simulink model "Monorail_Auxiliary_Power_Unit"  (R2021b)
settings: Solver=ode1  StartTime=0.0  StopTime=2.00  FixedStep=1e-06  MaxStep=1e-4  RelTol=1e-3
InitFcn:
  | %Input
  | V_supply_max = 910;
  | V_supply_min = 490;
  | V_supply_nom = 750;
  | R_supply = 1e-06;
  | L_in = 0.5e-03;
  | C_in = 215e-06;
  | R_Precharge = 1;
  | 
  | %PSFB_Voltage_Control
  | t_psfb_on = 0.05;
  | f_sw = 10e03;
  | V_dc_ref = 700;
  | V_dc_init = 450;
  | V_bat_ref = 24;
  | V_bat_init = 14;
  | Count_prd = 5000;
  | Half_prd = 2500;
  | Half_prd_fix = 2700;
  | Half_prd_var = 2300;
  | t_softstart = 100e-03;
  | Scale_factor_High = 1/737;
  | Scale_factor_Low = 1/48;
  | Kp_psfb = 2;
  | Ki_psfb =20;
  | Kp_feed = 0.00001;
  | PI_max = 1;
  | PI_min = 0;
  | t_enable = 1e-03;
  | Dead_prd = 1e-03
  | 
  | %PSFB_Current_Control
  | Scale_factor_i = 1/800;
  | I_cnst = 450;
  | I_over = 460;
  | Kp_psfb_i = 10;
  | Ki_psfb_i = 20;
  | 
  | %HF_Transformer
  | P_txf = 50e03;
  | f_txf = 10e03;
  | V_pri_txf = 1e03;
  | V_sec_high_txf = 720;
  | V_sec_low_txf = 27;
  | 
  | %DC_Link
  | L_filt = 1e-03;
  | C_filt = 215e-06;
  | R_Bleeder_700V = 0.5e03;
  | R_Bleeder_24V = 1e03
  | 
  | %Inverter_Control
  | t_inv_on = 1.5;
  | f_fund = 50;
  | V_phase_ref = 240;
  | Scale_factor_inv = 1/50e03;
  | Kp_inv = 0.05;
  | Ki_inv = 0.1;
  | PI_inv_max = 1;
  | PI_inv_min = -1;
  | I_Line_ref = 35;
  | Scale_factor_Iinv = 1/1e03;
  | Iinvov = 40;
  | Kp_Iinv = 0.05;
  | Ki_Iinv = 0.1;
  | t_dead = 2e-06;
  | 
  | %Inverter_Filter
  | L_sin_filt = 0.85e-03;
  | C_sin_filt = 30e-06;
  | 
  | %Zigzag
  | P_zigzag = 2.5e3;
  | f_zigzag = 50;
  | V_zigzag = 415;
  | 
  | %Load
  | R_load_750V = 6;
  | L_load_750V = 14.3e-03;
  | R_overload_750V = 6;
  | L_overload_750V = 14.3e-03;
  | t_overload_750V = 5;
  | R_load_24V = 53e-03;
  | R_overload_24V = 168e-03;
  | t_overload_24V = 5;
  | R_load_si = 24;
  | t_load_si = 10;
undefined symbols (not defined in the file): Ion, Lithium
libraries: spsSeriesRLCBranchLib x35, spsIGBTDiodeLib x14, spsDiodeLib x13, spsMeanLib x11, spsBreakerLib x9, spsVoltageMeasurementLib x9, simulink x8, spsRMSLib x8, spsCurrentMeasurementLib x6, dspfdesign x6, spsabctodq0Lib x4, spsLinearTransformerLib x2
(part 1 of 3)
settings Model: ModifiedByFormat=Sourjya_Mondal  Creator=Sourjya_Mondal  LastModifiedBy=Sourjya_Mondal
settings SolverCC: AlgebraicLoopSolver=TrustRegion  AutoInsertRateTranBlk=on
settings DataIOCC: ReturnWorkspaceOutputs=off
settings OptimizationCC: LifeSpan=inf
settings DebuggingCC: SFUnexpectedBacktrackingDiag=warning  SFNoUnconditionalDefaultTransitionDiag=warning  SFExecutionAtInitializationDiag=none  SFMachineParentedDataDiag=warning  ArithmeticOperatorsInVariantConditions=warning
settings SFSimCC: SimUseLocalCustomCode=off  CustomCodeUndefinedFunction=UseInterfaceOnly
settings RTWCC: RTWUseLocalCustomCode=off
settings CodeAppCC: StateflowObjectComments=on
settings GRTTargetCC: TargetLangStandard=C89/C90 (ANSI)
settings ConfigComp: CovMetricSettings=dw  CovSaveCumulativeToWorkspaceVar=on  CovSaveSingleToWorkspaceVar=on  CovExternalEMLEnable=off
settings SimscapeCC: SimscapeNormalizeSystem=off

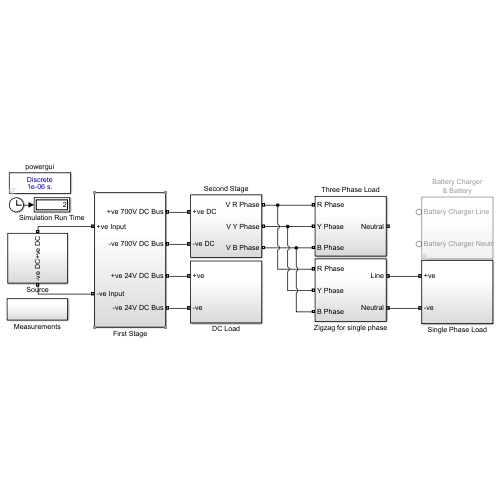
[thumbnail: Simulink's stored preview of the top-level diagram]
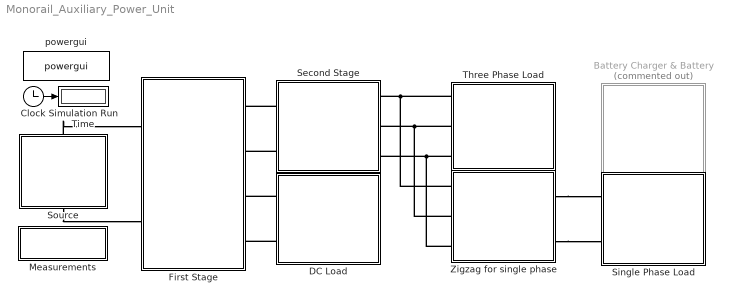
== system Monorail_Auxiliary_Power_Unit ==
  Battery Charger & Battery : Subsystem  Commented=on
  Clock : Clock
  DC Load : Subsystem
  First Stage : Subsystem
  Measurements : Subsystem
  Second Stage : Subsystem
  Simulation Run Time : Display
  Single Phase Load : Subsystem
  Source : Subsystem
  Three Phase Load : Subsystem
  Zigzag for single phase : Subsystem
  powergui : spspowerguiLib/powergui  Priority=1  SimulationMode=Discrete  SampleTime=1e-06  frequency=60  Iterations=50  frequencyindice=0  Pbase=100e6  ErrMax=1e-4  UnitsV=kV  UnitsW=MW  buscounter=0  FunctionMessages=off  echomessages=off  EnableUseOfTLC=off  CurrentSourceSwitches=off  DisableSnubberDevices=off  DisableRonSwitches=off  DisableVfSwitches=off  DisplayEquations=off  AutomaticDiscreteSolvers=off  SolverType=Tustin/Backward Euler (TBE)  Interpol=off  ExternalGateDelay=off  methode=off  Ts=100  x0status=blocks  SPID=on  SwTol=0  HookPort=off  NonlinearTolerance=1e-4  nMaxIteration=100  ContinueOnMaxIteration=off  RestoreLinks=warning  ResistiveCurrentMeasurement=off  Frange=[0:2:500]  Ylog=off  Xlog=on  ShowGrid=off  save=off  variable=ZData  structure=V_line  ZoomFFT=off  StartTime=0.1  cycles=5  DisplayStyle=1  fundamental=50  FreqAxis=off  MaxFrequency=10000  frequencyindicesteady=1  RmsSteady=1  display=off
  wires:
  Clock/1 -> Simulation Run Time/1
  connections:
  Source/LConn1 -- First Stage/LConn2
  Source/RConn1 -- First Stage/LConn1
  Second Stage/LConn1 -- First Stage/RConn1
  Second Stage/LConn2 -- First Stage/RConn2
  Three Phase Load/LConn1 -- Second Stage/RConn1 -- Zigzag for single phase/LConn1
  Three Phase Load/LConn3 -- Zigzag for single phase/LConn3 -- Second Stage/RConn3
  DC Load/LConn1 -- First Stage/RConn3
  DC Load/LConn2 -- First Stage/RConn4
  Three Phase Load/LConn2 -- Zigzag for single phase/LConn2 -- Second Stage/RConn2
  Zigzag for single phase/RConn1 -- Single Phase Load/LConn1
  Zigzag for single phase/RConn2 -- Single Phase Load/LConn2

== system Monorail_Auxiliary_Power_Unit/Battery Charger & Battery ==
  Battery : spsBatteryLib/Battery  BatType=Lithium-Ion  ShowTempParam=off  ThermalPreset=no  ShowAgeParam=off  NomV=24  NomQ=10  SOC=0  Batt_Tr=30  PresetModel=on  MaxQ=10  MinV=18  FullV=27.9357  Dis_rate=4.3478  R=0.024  Normal_OP=9.0435  expZone="[25.9293     0.491304]"  current=[6.5 13 32.5]  Units=Time  Tci=20  NomT=20  T2=-30  MaxQ2=4.8  FullV2=7.1  Normal_OP2=5.655  expZone2="[6.58           1]"  Rca=0.6  ti=2000  Dp=0  Neq0=0  Tsim=1e6  Ta1=25  Qeol=5.4*0.9  Reol=0.013333*1.2  Char_age=[2.3478, 3]  Dis_age=[2.3478, 10]  N1=1500  N2=10500  N3=1000  N4=1400  Ta2=45  N5=950
  Bus Selector : BusSelector  OutputSignals=Input Voltage (V),Input Current (A),Output Voltage (V),Output Current (A),Voltage limit (V),Current limit (A),Output KWh,Output Ah
  Bus Selector1 : BusSelector  OutputSignals=Voltage (V),Current (A),SOC (%)
  CCCV Battery Charger : electricdrivelib/Extra Sources/CCCV Battery Charger  Preset=Custom specifications  P_nom=800  s_type=1-phase AC  n_connect=off  eff_volt=240  in_freq=50  in_I_ripple=10  in_I_freq=1000  EFF_en=off  EFF_val=[0.627 0.803 0.855 0.871 0.872 0.864]  EFF_fu=[0.063 0.177 0.293 0.483 0.674 0.914]  THD_en=off  I_THD_val=[0.327 0.394 0.394 0.351 0.289 0.265]  I_THD_fu=[0.056 0.136 0.194 0.303 0.555 0.916]  H_DIST_rt=[0.199 1.297 0.328 0.029 0.416 0.200]  H_DIST_fr=[3 5 7 9 11 13]  PF_en=off  PF_val=[0.316 0.532 0.662 0.731 0.780 0.792]  PF_fu=[0.067 0.230 0.445 0.625 0.794 0.919]  Out_mode=Constant Current - Constant Voltage (CCCV)  DynInT=off  I_cst=10  V_cst=32  ABS_en=off  V_abs=142  ABS_end=Time based  ABS_time=3600  ABS_i=40  ripple=0.5  swF=1000  overshoot=1  stable_t=2  VoltComp=off  V_comp=-0.18  nom_temp=20
      settings: SourceProductBaseCode=PS
  Scope : Scope  NumInputPorts=8
  Scope1 : Scope  NumInputPorts=3
  Battery Charger Line : PMIOPort  Side=Left
  Battery Charger Neutral : PMIOPort  Port=2  Side=Left
  wires:
  Battery/1 -> Bus Selector1/1
  CCCV Battery Charger/1 -> Bus Selector/1
  Bus Selector/1 -> Scope/1  "<Input Voltage (V)>"
  Bus Selector/2 -> Scope/2  "<Input Current (A)>"
  Bus Selector/3 -> Scope/3  "<Output Voltage (V)>"
  Bus Selector/4 -> Scope/4  "<Output Current (A)>"
  Bus Selector/5 -> Scope/5  "<Voltage limit (V)>"
  Bus Selector/6 -> Scope/6  "<Current limit (A)>"
  Bus Selector/7 -> Scope/7  "<Output KWh>"
  Bus Selector/8 -> Scope/8  "<Output Ah>"
  Bus Selector1/1 -> Scope1/1, [VBat]  "<Voltage (V)>"
  Bus Selector1/2 -> [IBat], Scope1/2  "<Current (A)>"
  Bus Selector1/3 -> [Soc_Bt], Scope1/3  "<SOC (%)>"
  connections:
  Battery/LConn2 -- CCCV Battery Charger/RConn2
  CCCV Battery Charger/LConn2 -- Battery Charger Neutral/RConn1
  CCCV Battery Charger/LConn1 -- Battery Charger Line/RConn1
  Battery/LConn1 -- CCCV Battery Charger/RConn1

== system Monorail_Auxiliary_Power_Unit/DC Load ==
  Breaker : spsBreakerLib/Breaker  InitialState=0  SwitchingTimes="[1/60  5/60]"  External=on  BreakerResistance=0.01  SnubberResistance=1e6  SnubberCapacitance=inf  Measurements=None  MoreParameters=on  NoBreakLoop=off
      settings: SourceProductBaseCode=PS
  Enable : Step  Time=t_overload_24V  SampleTime=0
  Load 24V : spsSeriesRLCBranchLib/Series RLC Branch  LConnTagsString=__new0  RConnTagsString=__new0  BranchType=R  Resistance=R_load_24V  Inductance=1e-3  SetiL0=off  InitialCurrent=0  Capacitance=1e-6  Setx0=off  InitialVoltage=0  Measurements=None
  Overload 24V : spsSeriesRLCBranchLib/Series RLC Branch  LConnTagsString=__new0  RConnTagsString=__new0  BranchType=R  Resistance=R_overload_24V  Inductance=1e-3  SetiL0=off  InitialCurrent=0  Capacitance=1e-6  Setx0=off  InitialVoltage=0  Measurements=None
  +ve : PMIOPort  Side=Left
  -ve : PMIOPort  Port=2  Side=Left
  wires:
  Enable/1 -> Breaker/1
  connections:
  Load 24V/RConn1 -- -ve/RConn1 -- Overload 24V/RConn1
  Breaker/RConn1 -- Overload 24V/LConn1
  Load 24V/LConn1 -- +ve/RConn1 -- Breaker/LConn1

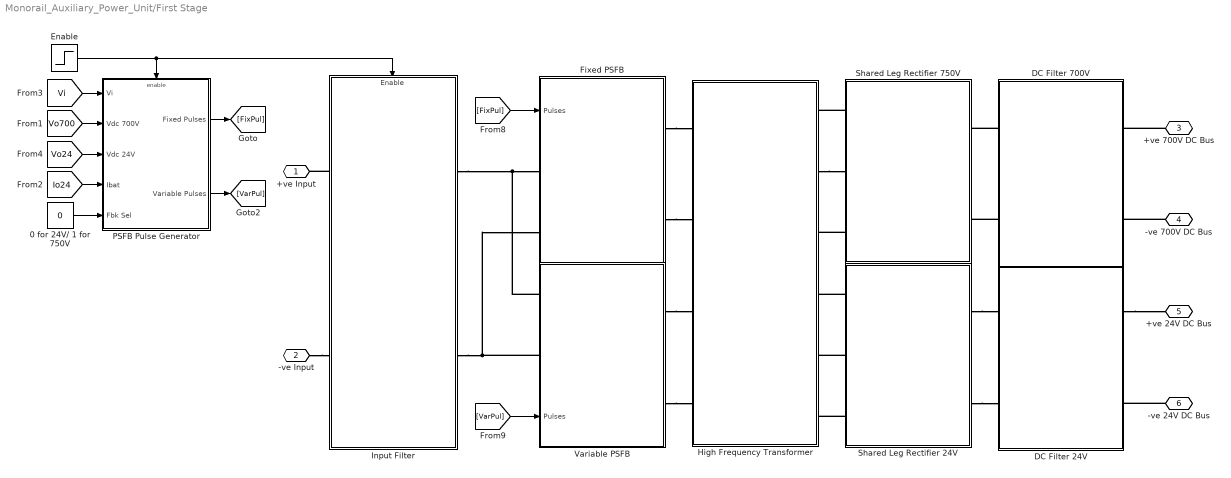
== system Monorail_Auxiliary_Power_Unit/First Stage ==
  0 for 24V/ 1 for 750V : Constant  Value=0
  DC Filter 24V : Subsystem
  DC Filter 700V : Subsystem
  Enable : Step  Time=t_psfb_on  SampleTime=0
  Fixed PSFB : Subsystem
  High Frequency Transformer : Subsystem
  Input Filter : Subsystem
      settings: PortSchema="{\"entries\":[{\"content\":{\"sides\":[{\"content\":{\"connectorIds\":[\"LConn1\",\"LConn2\"]},\"type\":\"ConnectorPlacement.EquallySpacedRectSide\",\"uuid\":\"355a31a2-ce4b-4446-9817-9663033cd28f\"},{\"content\":{\"connectorIds\":[\"RConn1\",\"RConn2\"],\"side\":\"RIGHT\"},\"type\":\"ConnectorPlacement.EquallySpacedRectSide\",\"uuid\":\"b1fa4b98-51e4-4b38-9334-3febb64d3166\"},{\"content\":{\"connectorIds\":[\"In1\"],\"side\":\"TOP\"},\"type\":\"ConnectorPlacement.EquallySpacedRectSide\",\"uuid\":\"3f1f76b0-45f3-4470-8606-701da3bcbe91\"}]},\"type\":\"ConnectorPlacement.EquallySpacedConnector\",\"uuid\":\"958f5b0f-2907-4940-ab6c-951926d8c97d\"}],\"packageUris\":[\"http://schema.mathworks.com/mf0/Connector/19700101\"],\"version\":\"1.0\"}"
  PSFB Pulse Generator : Subsystem
  Shared Leg Rectifier 24V : Subsystem
  Shared Leg Rectifier 750V : Subsystem
  Variable PSFB : Subsystem
      settings: PortSchema="{\"entries\":[{\"content\":{\"sides\":[{\"content\":{\"connectorIds\":[\"LConn1\",\"LConn2\",\"In1\"]},\"type\":\"ConnectorPlacement.EquallySpacedRectSide\",\"uuid\":\"164ee9a8-2883-4226-b641-75c923cc026a\"},{\"content\":{\"connectorIds\":[\"RConn1\",\"RConn2\"],\"side\":\"RIGHT\"},\"type\":\"ConnectorPlacement.EquallySpacedRectSide\",\"uuid\":\"3b4b1bb8-e497-4734-a92c-e609f39791cc\"},{\"content\":{\"connectorIds\":[],\"side\":\"TOP\"},\"type\":\"ConnectorPlacement.EquallySpacedRectSide\",\"uuid\":\"0bc5d7e7-4d54-414e-b6a1-3dfe739bfaa8\"}]},\"type\":\"ConnectorPlacement.EquallySpacedConnector\",\"uuid\":\"01def37e-b1d8-481f-9d3c-6964dbf0bd56\"}],\"packageUris\":[\"http://schema.mathworks.com/mf0/Connector/19700101\"],\"version\":\"1.0\"}"
  +ve Input : PMIOPort  Side=Left
  -ve Input : PMIOPort  Port=2  Side=Left
  +ve 700V DC Bus : PMIOPort  Port=3  Side=Right
  -ve 700V DC Bus : PMIOPort  Port=4  Side=Right
  +ve 24V DC Bus : PMIOPort  Port=5  Side=Right
  -ve 24V DC Bus : PMIOPort  Port=6  Side=Right
  wires:
  [FixPul] -> Fixed PSFB/1(Pulses)
  [VarPul] -> Variable PSFB/1(Pulses)
  0 for 24V/ 1 for 750V/1 -> PSFB Pulse Generator/5(Fbk Sel)
  PSFB Pulse Generator/1(Fixed Pulses) -> [FixPul]
  PSFB Pulse Generator/2(Variable Pulses) -> [VarPul]
  Enable/1 -> Input Filter/1(Enable), PSFB Pulse Generator/Enable
  [Vo24] -> PSFB Pulse Generator/3(Vdc 24V)
  [Vo700] -> PSFB Pulse Generator/2(Vdc 700V)
  [Io24] -> PSFB Pulse Generator/4(Ibat)
  [Vi] -> PSFB Pulse Generator/1(Vi)
  connections:
  Shared Leg Rectifier 24V/LConn2 -- High Frequency Transformer/RConn5
  Shared Leg Rectifier 24V/LConn1 -- High Frequency Transformer/RConn4
  +ve 700V DC Bus/RConn1 -- DC Filter 700V/RConn1
  Shared Leg Rectifier 24V/RConn1 -- DC Filter 24V/LConn1
  DC Filter 700V/LConn2 -- Shared Leg Rectifier 750V/RConn2
  Shared Leg Rectifier 24V/RConn2 -- DC Filter 24V/LConn2
  -ve 700V DC Bus/RConn1 -- DC Filter 700V/RConn2
  Shared Leg Rectifier 24V/LConn3 -- High Frequency Transformer/RConn6
  Fixed PSFB/RConn1 -- High Frequency Transformer/LConn1
  Fixed PSFB/RConn2 -- High Frequency Transformer/LConn2
  High Frequency Transformer/RConn2 -- Shared Leg Rectifier 750V/LConn2
  Shared Leg Rectifier 750V/LConn1 -- High Frequency Transformer/RConn1
  Variable PSFB/RConn1 -- High Frequency Transformer/LConn3
  Shared Leg Rectifier 750V/LConn3 -- High Frequency Transformer/RConn3
  Variable PSFB/RConn2 -- High Frequency Transformer/LConn4
  DC Filter 700V/LConn1 -- Shared Leg Rectifier 750V/RConn1
  -ve 24V DC Bus/RConn1 -- DC Filter 24V/RConn2
  DC Filter 24V/RConn1 -- +ve 24V DC Bus/RConn1
  Input Filter/RConn1 -- Variable PSFB/LConn1 -- Fixed PSFB/LConn1
  Input Filter/RConn2 -- Fixed PSFB/LConn2 -- Variable PSFB/LConn2
  -ve Input/RConn1 -- Input Filter/LConn2
  Input Filter/LConn1 -- +ve Input/RConn1

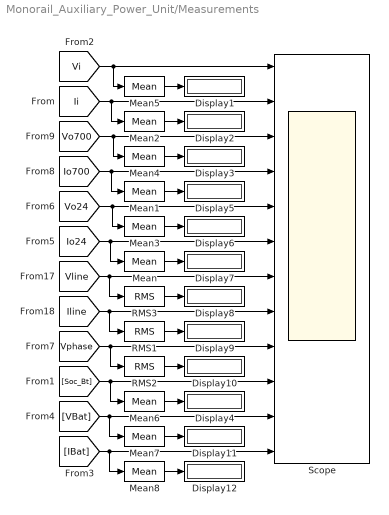
== system Monorail_Auxiliary_Power_Unit/Measurements ==
  Display{1..12} (12 alike) : Display
  Mean{,1..8} (9 alike) : spsMeanLib/Mean  Freq=f_fund  Vinit=0  Ts=0
  RMS1 : spsRMSLib/RMS  TrueRMS=on  Freq=f_fund  RMSInit=0  Ts=0
  RMS2 : spsRMSLib/RMS  TrueRMS=on  Freq=f_fund  RMSInit=0  Ts=0
  RMS3 : spsRMSLib/RMS  TrueRMS=on  Freq=f_fund  RMSInit=0  Ts=0
  Scope : Scope  NumInputPorts=12
  wires:
  Mean4/1 -> Display3/1
  [Io24] -> Mean/1, Scope/6
  Mean/1 -> Display7/1
  RMS2/1 -> Display10/1
  [Ii] -> Mean2/1, Scope/2
  [Io700] -> Mean1/1, Scope/4
  [Vline] -> RMS3/1, Scope/7
  [Vi] -> Mean5/1, Scope/1
  [Vo24] -> Mean3/1, Scope/5
  [Vo700] -> Mean4/1, Scope/3
  Mean2/1 -> Display2/1
  Mean3/1 -> Display6/1
  Mean5/1 -> Display1/1
  [Iline] -> RMS1/1, Scope/8
  RMS3/1 -> Display8/1
  RMS1/1 -> Display9/1
  [Vphase] -> RMS2/1, Scope/9
  Mean1/1 -> Display5/1
  Mean6/1 -> Display4/1
  [Soc_Bt] -> Mean6/1, Scope/10
  [VBat] -> Mean7/1, Scope/11
  Mean7/1 -> Display11/1
  Mean8/1 -> Display12/1
  [IBat] -> Mean8/1, Scope/12

== system Monorail_Auxiliary_Power_Unit/Second Stage ==
  3 Phase Inverter : Subsystem
      settings: PortSchema="{\"entries\":[{\"content\":{\"sides\":[{\"content\":{\"connectorIds\":[\"LConn1\",\"LConn2\",\"LConn3\"]},\"type\":\"ConnectorPlacement.EquallySpacedRectSide\",\"uuid\":\"8e7d0507-4c36-4782-8146-44468d669e3a\"},{\"content\":{\"connectorIds\":[\"RConn1\",\"RConn2\"],\"side\":\"RIGHT\"},\"type\":\"ConnectorPlacement.EquallySpacedRectSide\",\"uuid\":\"09e1e120-4fd8-49b7-b722-b9eb2381e368\"},{\"content\":{\"connectorIds\":[\"In1\"],\"side\":\"TOP\"},\"type\":\"ConnectorPlacement.EquallySpacedRectSide\",\"uuid\":\"7de3d764-ed32-4b0a-aa2a-06a93e2fe6c9\"}]},\"type\":\"ConnectorPlacement.EquallySpacedConnector\",\"uuid\":\"5bdb4caa-516f-480e-aa48-8e9ce05b05aa\"}],\"packageUris\":[\"http://schema.mathworks.com/mf0/Connector/19700101\"],\"version\":\"1.0\"}"
  Enable : Step  Time=t_inv_on  SampleTime=0
  Input Breaker : Subsystem
      settings: PortSchema="{\"entries\":[{\"content\":{\"sides\":[{\"content\":{\"connectorIds\":[\"LConn1\",\"LConn2\"]},\"type\":\"ConnectorPlacement.EquallySpacedRectSide\",\"uuid\":\"164ee9a8-2883-4226-b641-75c923cc026a\"},{\"content\":{\"connectorIds\":[\"RConn1\",\"RConn2\"],\"side\":\"RIGHT\"},\"type\":\"ConnectorPlacement.EquallySpacedRectSide\",\"uuid\":\"3b4b1bb8-e497-4734-a92c-e609f39791cc\"},{\"content\":{\"connectorIds\":[\"In1\"],\"side\":\"TOP\"},\"type\":\"ConnectorPlacement.EquallySpacedRectSide\",\"uuid\":\"0bc5d7e7-4d54-414e-b6a1-3dfe739bfaa8\"}]},\"type\":\"ConnectorPlacement.EquallySpacedConnector\",\"uuid\":\"01def37e-b1d8-481f-9d3c-6964dbf0bd56\"}],\"packageUris\":[\"http://schema.mathworks.com/mf0/Connector/19700101\"],\"version\":\"1.0\"}"
  Pulse Generator : Subsystem
  Sine Filter : Subsystem
      settings: PortSchema="{\"entries\":[{\"content\":{\"sides\":[{\"content\":{\"connectorIds\":[\"LConn1\",\"LConn2\",\"LConn3\"]},\"type\":\"ConnectorPlacement.EquallySpacedRectSide\",\"uuid\":\"007b0c32-aad9-45d1-835d-643ed93e4465\"},{\"content\":{\"connectorIds\":[\"RConn1\",\"RConn2\",\"RConn3\"],\"side\":\"RIGHT\"},\"type\":\"ConnectorPlacement.EquallySpacedRectSide\",\"uuid\":\"5580f04d-d874-403c-95d7-850705f3d46b\"},{\"content\":{\"connectorIds\":[\"Out1\",\"Out2\"],\"side\":\"TOP\"},\"type\":\"ConnectorPlacement.EquallySpacedRectSide\",\"uuid\":\"34ef45c5-954c-4c95-874b-bb304e8a67b4\"}]},\"type\":\"ConnectorPlacement.EquallySpacedConnector\",\"uuid\":\"b06ae3f5-1afb-4356-b523-0824140ca574\"}],\"packageUris\":[\"http://schema.mathworks.com/mf0/Connector/19700101\"],\"version\":\"1.0\"}"
  +ve DC : PMIOPort  Side=Left
  -ve DC : PMIOPort  Port=2  Side=Left
  V R Phase : PMIOPort  Port=3  Side=Right
  V Y Phase : PMIOPort  Port=4  Side=Right
  V B Phase : PMIOPort  Port=5  Side=Right
  wires:
  Sine Filter/2(Vline) -> Pulse Generator/1(V feedback)
  Pulse Generator/1(Pulses) -> 3 Phase Inverter/1(Pulses)
  Enable/1 -> Input Breaker/1(Enable), Pulse Generator/Enable
  Sine Filter/1(Iline) -> Pulse Generator/2(I feedback)
  connections:
  V Y Phase/RConn1 -- Sine Filter/RConn2
  Sine Filter/LConn1 -- 3 Phase Inverter/LConn1
  Sine Filter/LConn3 -- 3 Phase Inverter/LConn3
  V B Phase/RConn1 -- Sine Filter/RConn3
  Sine Filter/LConn2 -- 3 Phase Inverter/LConn2
  V R Phase/RConn1 -- Sine Filter/RConn1
  Input Breaker/RConn1 -- 3 Phase Inverter/RConn1
  Input Breaker/LConn1 -- +ve DC/RConn1
  Input Breaker/RConn2 -- 3 Phase Inverter/RConn2
  Input Breaker/LConn2 -- -ve DC/RConn1

== system Monorail_Auxiliary_Power_Unit/Single Phase Load ==
  Breaker : spsBreakerLib/Breaker  InitialState=0  SwitchingTimes="[1/60  5/60]"  External=on  BreakerResistance=0.01  SnubberResistance=1e6  SnubberCapacitance=inf  Measurements=None  MoreParameters=on  NoBreakLoop=off
      settings: SourceProductBaseCode=PS
  Enable : Step  Time=t_load_si  SampleTime=0
  Single Phase 10A Load : spsSeriesRLCBranchLib/Series RLC Branch  LConnTagsString=__new0  RConnTagsString=__new0  BranchType=R  Resistance=R_load_si  Inductance=1e-3  SetiL0=off  InitialCurrent=0  Capacitance=1e-6  Setx0=off  InitialVoltage=0  Measurements=None
  +ve : PMIOPort  Side=Left
  -ve : PMIOPort  Port=2  Side=Left
  wires:
  Enable/1 -> Breaker/1
  connections:
  Breaker/LConn1 -- +ve/RConn1
  Breaker/RConn1 -- Single Phase 10A Load/LConn1
  Single Phase 10A Load/RConn1 -- -ve/RConn1

== system Monorail_Auxiliary_Power_Unit/Source ==
  Constant1 : Constant  Value=900
  R Source : spsSeriesRLCBranchLib/Series RLC Branch  LConnTagsString=__new0  RConnTagsString=__new0  BranchType=R  Resistance=R_supply  Inductance=0.5e-3  SetiL0=off  InitialCurrent=0  Capacitance=1e-6  Setx0=off  InitialVoltage=0  Measurements=None
  Saturation : Saturate  UpperLimit=V_supply_max  LowerLimit=V_supply_min
  V Supply : spsControlledVoltageSourceLib/Controlled Voltage Source  Initialize=on  Source_Type=DC  Amplitude=0  Phase=0  Frequency=0  Measurements=None
  +ve DC : PMIOPort  Side=Right
  -ve DC : PMIOPort  Port=2  Side=Left
  wires:
  Constant1/1 -> Saturation/1
  Saturation/1 -> V Supply/1
  connections:
  R Source/RConn1 -- +ve DC/RConn1
  V Supply/LConn1 -- -ve DC/RConn1
  V Supply/RConn1 -- R Source/LConn1

== system Monorail_Auxiliary_Power_Unit/Three Phase Load ==
  Breaker{,1..3} (4 alike) : spsBreakerLib/Breaker  InitialState=0  SwitchingTimes="[1/60  5/60]"  External=on  BreakerResistance=0.01  SnubberResistance=1e6  SnubberCapacitance=inf  Measurements=None  MoreParameters=on  NoBreakLoop=off
      settings: SourceProductBaseCode=PS
  L Load B : spsSeriesRLCBranchLib/Series RLC Branch  LConnTagsString=__new0  RConnTagsString=__new0  BranchType=L  Resistance=1  Inductance=L_load_750V  SetiL0=off  InitialCurrent=0  Capacitance=1e-6  Setx0=off  InitialVoltage=0  Measurements=None
  L Load R : spsSeriesRLCBranchLib/Series RLC Branch  LConnTagsString=__new0  RConnTagsString=__new0  BranchType=L  Resistance=1  Inductance=L_load_750V  SetiL0=off  InitialCurrent=0  Capacitance=1e-6  Setx0=off  InitialVoltage=0  Measurements=None
  L Load Y : spsSeriesRLCBranchLib/Series RLC Branch  LConnTagsString=__new0  RConnTagsString=__new0  BranchType=L  Resistance=1  Inductance=L_load_750V  SetiL0=off  InitialCurrent=0  Capacitance=1e-6  Setx0=off  InitialVoltage=0  Measurements=None
  L Overload B : spsSeriesRLCBranchLib/Series RLC Branch  LConnTagsString=__new0  RConnTagsString=__new0  BranchType=L  Resistance=1  Inductance=L_overload_750V  SetiL0=off  InitialCurrent=0  Capacitance=1e-6  Setx0=off  InitialVoltage=0  Measurements=None
  L Overload R : spsSeriesRLCBranchLib/Series RLC Branch  LConnTagsString=__new0  RConnTagsString=__new0  BranchType=L  Resistance=1  Inductance=L_overload_750V  SetiL0=off  InitialCurrent=0  Capacitance=1e-6  Setx0=off  InitialVoltage=0  Measurements=None
  L Overload Y : spsSeriesRLCBranchLib/Series RLC Branch  LConnTagsString=__new0  RConnTagsString=__new0  BranchType=L  Resistance=1  Inductance=L_overload_750V  SetiL0=off  InitialCurrent=0  Capacitance=1e-6  Setx0=off  InitialVoltage=0  Measurements=None
  R Load B : spsSeriesRLCBranchLib/Series RLC Branch  LConnTagsString=__new0  RConnTagsString=__new0  BranchType=R  Resistance=R_load_750V  Inductance=1e-3  SetiL0=off  InitialCurrent=0  Capacitance=1e-6  Setx0=off  InitialVoltage=0  Measurements=None
  R Load R : spsSeriesRLCBranchLib/Series RLC Branch  LConnTagsString=__new0  RConnTagsString=__new0  BranchType=R  Resistance=R_load_750V  Inductance=1e-3  SetiL0=off  InitialCurrent=0  Capacitance=1e-6  Setx0=off  InitialVoltage=0  Measurements=None
  R Load Y : spsSeriesRLCBranchLib/Series RLC Branch  LConnTagsString=__new0  RConnTagsString=__new0  BranchType=R  Resistance=R_load_750V  Inductance=1e-3  SetiL0=off  InitialCurrent=0  Capacitance=1e-6  Setx0=off  InitialVoltage=0  Measurements=None
  R Overload B : spsSeriesRLCBranchLib/Series RLC Branch  LConnTagsString=__new0  RConnTagsString=__new0  BranchType=R  Resistance=R_overload_750V  Inductance=1e-3  SetiL0=off  InitialCurrent=0  Capacitance=1e-6  Setx0=off  InitialVoltage=0  Measurements=None
  R Overload R : spsSeriesRLCBranchLib/Series RLC Branch  LConnTagsString=__new0  RConnTagsString=__new0  BranchType=R  Resistance=R_overload_750V  Inductance=1e-3  SetiL0=off  InitialCurrent=0  Capacitance=1e-6  Setx0=off  InitialVoltage=0  Measurements=None
  R Overload Y : spsSeriesRLCBranchLib/Series RLC Branch  LConnTagsString=__new0  RConnTagsString=__new0  BranchType=R  Resistance=R_overload_750V  Inductance=1e-3  SetiL0=off  InitialCurrent=0  Capacitance=1e-6  Setx0=off  InitialVoltage=0  Measurements=None
  Step : Step  Time=t_overload_750V  SampleTime=0
  R Phase : PMIOPort  Side=Left
  Y Phase : PMIOPort  Port=2  Side=Left
  B Phase : PMIOPort  Port=3  Side=Left
  Neutral : PMIOPort  Port=4  Side=Right
  wires:
  Step/1 -> Breaker/1, Breaker1/1, Breaker2/1, Breaker3/1
  connections:
  R Load B/LConn1 -- B Phase/RConn1 -- Breaker2/LConn1
  R Load Y/LConn1 -- Y Phase/RConn1 -- Breaker1/LConn1
  R Load R/LConn1 -- R Phase/RConn1 -- Breaker/LConn1
  R Load B/RConn1 -- L Load B/LConn1
  L Overload R/RConn1 -- L Overload B/RConn1 -- L Overload Y/RConn1 -- Breaker3/LConn1
  L Overload Y/LConn1 -- R Overload Y/RConn1
  L Overload R/LConn1 -- R Overload R/RConn1
  R Overload R/LConn1 -- Breaker/RConn1
  L Overload B/LConn1 -- R Overload B/RConn1
  R Overload B/LConn1 -- Breaker2/RConn1
  R Overload Y/LConn1 -- Breaker1/RConn1
  R Load R/RConn1 -- L Load R/LConn1
  L Load B/RConn1 -- Breaker3/RConn1 -- Neutral/RConn1 -- L Load R/RConn1 -- L Load Y/RConn1
  L Load Y/LConn1 -- R Load Y/RConn1

== system Monorail_Auxiliary_Power_Unit/Zigzag for single phase ==
  "Grounding Transformer " : spsGroundingTransformerLib/Grounding Transformer   UNITS=SI  NominalPower=[P_zigzag f_zigzag]  NominalVoltage=V_zigzag  ZeroSequenceImpedance_pu=[0.025 0.75]  MagnetizationBranch_pu=[500 500]  ZeroSequenceImpedance_SI=[1.7223 51.668]  MagnetizationBranch_SI=[34445 34445]  Measurements=None
      settings: SourceProductBaseCode=PS
  Mux : Mux  Inputs=3
  Voltage Measurement : spsVoltageMeasurementLib/Voltage Measurement  PhasorSimulation=off  OutputType=Complex  PSBequivalent=0
  Voltage Measurement1 : spsVoltageMeasurementLib/Voltage Measurement  PhasorSimulation=off  OutputType=Complex  PSBequivalent=0
  Voltage Measurement2 : spsVoltageMeasurementLib/Voltage Measurement  PhasorSimulation=off  OutputType=Complex  PSBequivalent=0
  R Phase : PMIOPort  Side=Left
  Y Phase : PMIOPort  Port=2  Side=Left
  B Phase : PMIOPort  Port=3  Side=Left
  Line : PMIOPort  Port=4  Side=Right
  Neutral : PMIOPort  Port=5  Side=Right
  tag scope: Vphase=global
  wires:
  Voltage Measurement/1 -> Mux/1
  Mux/1 -> [Vphase]
  Voltage Measurement2/1 -> Mux/3
  Voltage Measurement1/1 -> Mux/2
  connections:
  Neutral/RConn1 -- "Grounding Transformer "/RConn1 -- Voltage Measurement/LConn2 -- Voltage Measurement1/LConn2 -- Voltage Measurement2/LConn2
  "Grounding Transformer "/LConn1 -- Line/RConn1 -- Voltage Measurement/LConn1 -- R Phase/RConn1
  Y Phase/RConn1 -- Voltage Measurement1/LConn1 -- "Grounding Transformer "/LConn2
  B Phase/RConn1 -- Voltage Measurement2/LConn1 -- "Grounding Transformer "/LConn3

== system Monorail_Auxiliary_Power_Unit/First Stage/DC Filter 24V ==
  C Filter 24V : spsSeriesRLCBranchLib/Series RLC Branch  LConnTagsString=__new0  RConnTagsString=__new0  BranchType=C  Resistance=12.25  Inductance=1e-3  SetiL0=off  InitialCurrent=0  Capacitance=C_filt  Setx0=off  InitialVoltage=0  Measurements=None
  Diode : spsDiodeLib/Diode  Ron=0.001  Lon=0  Vf=0.8  IC=0  UseSnubber=0  Rs=500  Cs=250e-9  Measurements=off
  Iout 24V : spsCurrentMeasurementLib/Current Measurement  PhasorSimulation=off  OutputType=Complex  PSBequivalent=0
  L Filter 24V : spsSeriesRLCBranchLib/Series RLC Branch  LConnTagsString=__new0  RConnTagsString=__new0  BranchType=L  Resistance=12.25  Inductance=L_filt  SetiL0=off  InitialCurrent=0  Capacitance=1e-6  Setx0=off  InitialVoltage=0  Measurements=None
  R Bleed 24V : spsSeriesRLCBranchLib/Series RLC Branch  LConnTagsString=__new0  RConnTagsString=__new0  BranchType=R  Resistance=R_Bleeder_24V  Inductance=1e-3  SetiL0=off  InitialCurrent=0  Capacitance=1e-6  Setx0=off  InitialVoltage=0  Measurements=None
  Vout 24V : spsVoltageMeasurementLib/Voltage Measurement  PhasorSimulation=off  OutputType=Complex  PSBequivalent=0
  +ve Filter In : PMIOPort  Side=Left
  -ve Filter In : PMIOPort  Port=2  Side=Left
  +ve Filter Out : PMIOPort  Port=3  Side=Right
  -ve Filter Out : PMIOPort  Port=4  Side=Right
  tag scope: Io24=global, Vo24=global
  wires:
  Vout 24V/1 -> [Vo24]
  Iout 24V/1 -> [Io24]
  connections:
  Vout 24V/LConn2 -- R Bleed 24V/RConn1 -- -ve Filter In/RConn1 -- C Filter 24V/RConn1 -- -ve Filter Out/RConn1
  Vout 24V/LConn1 -- Diode/RConn1 -- Iout 24V/LConn1
  L Filter 24V/RConn1 -- +ve Filter In/RConn1
  Iout 24V/RConn1 -- +ve Filter Out/RConn1
  R Bleed 24V/LConn1 -- Diode/LConn1 -- L Filter 24V/LConn1 -- C Filter 24V/LConn1

== system Monorail_Auxiliary_Power_Unit/First Stage/DC Filter 700V ==
  C Filter 750V : spsSeriesRLCBranchLib/Series RLC Branch  LConnTagsString=__new0  RConnTagsString=__new0  BranchType=C  Resistance=12.25  Inductance=1e-3  SetiL0=off  InitialCurrent=0  Capacitance=C_filt  Setx0=off  InitialVoltage=0  Measurements=None
  Chopper : Subsystem  Commented=on
  IGBT : spsIGBTLib/IGBT  Commented=on  Ron=0.001  Lon=0  Vf=1  Tf=1e-6  Tt=2e-6  IC=0  Rs=1e5  Cs=inf  Measurements=on
  Iout 700V : spsCurrentMeasurementLib/Current Measurement  PhasorSimulation=off  OutputType=Complex  PSBequivalent=0
  L Filter 700V : spsSeriesRLCBranchLib/Series RLC Branch  LConnTagsString=__new0  RConnTagsString=__new0  BranchType=L  Resistance=12.25  Inductance=L_filt  SetiL0=off  InitialCurrent=0  Capacitance=1e-6  Setx0=off  InitialVoltage=0  Measurements=None
  R Bleed 700V : spsSeriesRLCBranchLib/Series RLC Branch  LConnTagsString=__new0  RConnTagsString=__new0  BranchType=R  Resistance=R_Bleeder_700V  Inductance=1e-3  SetiL0=off  InitialCurrent=0  Capacitance=1e-6  Setx0=off  InitialVoltage=0  Measurements=None
  Scope2 : Scope  Commented=on
  Vout 700V : spsVoltageMeasurementLib/Voltage Measurement  PhasorSimulation=off  OutputType=Complex  PSBequivalent=0
  +ve Filter In : PMIOPort  Side=Left
  -ve Filter In : PMIOPort  Port=2  Side=Left
  +ve Filter Out : PMIOPort  Port=3  Side=Right
  -ve Filter Out : PMIOPort  Port=4  Side=Right
  tag scope: Io700=global, Vo700=global
  wires:
  Vout 700V/1 -> [Vo700]
  Iout 700V/1 -> [Io700]
  IGBT/1 -> Scope2/1
  Chopper/1(Chopper Pulse) -> IGBT/1
  connections:
  +ve Filter In/RConn1 -- L Filter 700V/RConn1
  Iout 700V/RConn1 -- +ve Filter Out/RConn1
  C Filter 750V/RConn1 -- Vout 700V/LConn2 -- -ve Filter Out/RConn1 -- R Bleed 700V/RConn1 -- -ve Filter In/RConn1
  L Filter 700V/LConn1 -- C Filter 750V/LConn1 -- R Bleed 700V/LConn1 -- Vout 700V/LConn1 -- Iout 700V/LConn1

== system Monorail_Auxiliary_Power_Unit/First Stage/Fixed PSFB ==
  Pulses : Inport
  Demux : Demux  Outputs=2
  IGBT/Diode{,1..3} (4 alike) : spsIGBTDiodeLib/IGBT//Diode  Ron=1e-3  Rs=1e5  Cs=inf  Measurements=on
  Scope{1..3,5} (4 alike) : Scope  Commented=on
  +ve : PMIOPort  Side=Left
  -ve : PMIOPort  Port=2  Side=Left
  Line : PMIOPort  Port=3  Side=Right
  Neutral : PMIOPort  Port=4  Side=Right
  wires:
  [RTop] -> IGBT/Diode/1
  [RTop] -> IGBT/Diode3/1
  [YTop] -> IGBT/Diode1/1
  [YTop] -> IGBT/Diode2/1
  Demux/1 -> [RTop]
  Demux/2 -> [YTop]
  Pulses/1 -> Demux/1
  IGBT/Diode/1 -> Scope5/1
  IGBT/Diode1/1 -> Scope1/1
  IGBT/Diode2/1 -> Scope2/1
  IGBT/Diode3/1 -> Scope3/1
  connections:
  IGBT/Diode2/RConn1 -- IGBT/Diode3/LConn1 -- Neutral/RConn1
  IGBT/Diode/RConn1 -- Line/RConn1 -- IGBT/Diode1/LConn1
  IGBT/Diode/LConn1 -- +ve/RConn1 -- IGBT/Diode2/LConn1
  IGBT/Diode1/RConn1 -- -ve/RConn1 -- IGBT/Diode3/RConn1

== system Monorail_Auxiliary_Power_Unit/First Stage/High Frequency Transformer ==
  Linear Transformer : spsLinearTransformerLib/Linear Transformer  UNITS=SI  NominalPower=[P_txf f_txf]  winding1=[V_pri_txf 0 0]  winding2=[V_sec_high_txf 0 0]  ThreeWindings=on  winding3=[V_sec_low_txf 0 0]  RmLm=[inf inf]  Measurements=None  DataType=on
  Linear Transformer1 : spsLinearTransformerLib/Linear Transformer  UNITS=SI  NominalPower=[P_txf f_txf]  winding1=[V_pri_txf 0 0]  winding2=[V_sec_high_txf 0 0]  ThreeWindings=on  winding3=[V_sec_low_txf 0 0]  RmLm=[inf inf]  Measurements=None  DataType=on
  FixPSFB Line : PMIOPort  Side=Left
  FixPSFB Neutral : PMIOPort  Port=2  Side=Left
  VarPSFB Neutral : PMIOPort  Port=3  Side=Left
  VarPSFB Line : PMIOPort  Port=4  Side=Left
  750V R : PMIOPort  Port=5  Side=Right
  750V Y : PMIOPort  Port=6  Side=Right
  750V B : PMIOPort  Port=7  Side=Right
  24V R : PMIOPort  Port=8  Side=Right
  24V Y : PMIOPort  Port=9  Side=Right
  24V B : PMIOPort  Port=10  Side=Right
  connections:
  FixPSFB Line/RConn1 -- Linear Transformer/LConn1
  Linear Transformer/RConn1 -- 750V Y/RConn1
  Linear Transformer/RConn4 -- Linear Transformer1/RConn4 -- 24V R/RConn1
  750V R/RConn1 -- Linear Transformer/RConn2 -- Linear Transformer1/RConn2
  24V Y/RConn1 -- Linear Transformer1/RConn3
  VarPSFB Neutral/RConn1 -- Linear Transformer1/LConn2
  750V B/RConn1 -- Linear Transformer1/RConn1
  VarPSFB Line/RConn1 -- Linear Transformer1/LConn1
  FixPSFB Neutral/RConn1 -- Linear Transformer/LConn2
  24V B/RConn1 -- Linear Transformer/RConn3

== system Monorail_Auxiliary_Power_Unit/First Stage/Input Filter ==
  Enable : Inport
  Breaker : spsBreakerLib/Breaker  InitialState=0  SwitchingTimes="[1/60  5/60]"  External=on  BreakerResistance=R_supply  SnubberResistance=1e6  SnubberCapacitance=inf  Measurements=None  MoreParameters=on  NoBreakLoop=off
      settings: SourceProductBaseCode=PS
  C1 Input : spsSeriesRLCBranchLib/Series RLC Branch  LConnTagsString=__new0  RConnTagsString=__new0  BranchType=C  Resistance=0.1  Inductance=1e-3  SetiL0=off  InitialCurrent=0  Capacitance=C_in  Setx0=off  InitialVoltage=0  Measurements=None
  C2 Input : spsSeriesRLCBranchLib/Series RLC Branch  LConnTagsString=__new0  RConnTagsString=__new0  BranchType=C  Resistance=12.25  Inductance=1e-3  SetiL0=off  InitialCurrent=0  Capacitance=C_in  Setx0=off  InitialVoltage=0  Measurements=None
  Iin : spsCurrentMeasurementLib/Current Measurement  PhasorSimulation=off  OutputType=Complex  PSBequivalent=0
  L Input : spsSeriesRLCBranchLib/Series RLC Branch  LConnTagsString=__new0  RConnTagsString=__new0  BranchType=L  Resistance=12.25  Inductance=L_in  SetiL0=off  InitialCurrent=0  Capacitance=1e-6  Setx0=off  InitialVoltage=0  Measurements=None
  Pre-Charge Resistor : spsSeriesRLCBranchLib/Series RLC Branch  LConnTagsString=__new0  RConnTagsString=__new0  BranchType=R  Resistance=R_Precharge  Inductance=1e-3  SetiL0=off  InitialCurrent=0  Capacitance=1e-6  Setx0=off  InitialVoltage=0  Measurements=None
  Vin : spsVoltageMeasurementLib/Voltage Measurement  PhasorSimulation=off  OutputType=Complex  PSBequivalent=0
  +ve Filter In : PMIOPort  Side=Left
  -ve Filter In : PMIOPort  Port=2  Side=Left
  +ve Filter out : PMIOPort  Port=3  Side=Right
  -ve Filter out : PMIOPort  Port=4  Side=Right
  tag scope: Ii=global, Vi=global
  wires:
  Vin/1 -> [Vi]
  Iin/1 -> [Ii]
  Enable/1 -> Breaker/1
  connections:
  C1 Input/LConn1 -- L Input/LConn1 -- Iin/RConn1
  C1 Input/RConn1 -- -ve Filter out/RConn1 -- C2 Input/RConn1 -- Vin/LConn2 -- -ve Filter In/RConn1
  L Input/RConn1 -- +ve Filter out/RConn1 -- C2 Input/LConn1
  Vin/LConn1 -- Pre-Charge Resistor/RConn1 -- Iin/LConn1 -- Breaker/RConn1
  Breaker/LConn1 -- Pre-Charge Resistor/LConn1 -- +ve Filter In/RConn1

== system Monorail_Auxiliary_Power_Unit/First Stage/PSFB Pulse Generator ==
  Vi : Inport
  Vdc 700V : Inport  Port=2
  Vdc 24V : Inport  Port=3
  Ibat : Inport  Port=4
  Fbk Sel : Inport  Port=5
  Enable : EnablePort
  Current Loop : Subsystem
      settings: PortSchema="{\"entries\":[{\"content\":{\"sides\":[{\"content\":{\"connectorIds\":[\"In1\"]},\"type\":\"ConnectorPlacement.EquallySpacedRectSide\",\"uuid\":\"3301e0b6-592f-4625-8269-e8a7d97e22bd\"},{\"content\":{\"connectorIds\":[\"Out1\",\"Out2\"],\"side\":\"RIGHT\"},\"type\":\"ConnectorPlacement.EquallySpacedRectSide\",\"uuid\":\"054d50bd-24b4-4709-a51e-c662b2406f8c\"},{\"content\":{\"connectorIds\":[],\"side\":\"TOP\"},\"type\":\"ConnectorPlacement.EquallySpacedRectSide\",\"uuid\":\"f115f2c5-740b-4df4-bc67-82446fee67ee\"},{\"content\":{\"connectorIds\":[\"Out3\"],\"side\":\"BOTTOM\"},\"type\":\"ConnectorPlacement.EquallySpacedRectSide\",\"uuid\":\"dcd527d4-e1a8-4b7f-b912-8b04fa46b01b\"}]},\"type\":\"ConnectorPlacement.EquallySpacedConnector\",\"uuid\":\"b1a80dea-a418-49d9-810f-d923c5601f97\"}],\"packageUris\":[\"http://schema.mathworks.com/mf0/Connector/19700101\"],\"version\":\"1.0\"}"
  Loop Select : Subsystem
  Voltage Loop : Subsystem
  Fixed Pulses : Outport
  Variable Pulses : Outport  Port=2
  wires:
  Ibat/1 -> Current Loop/1(Ibat)
  Vdc 700V/1 -> Voltage Loop/2(Vo 700V)
  Vdc 24V/1 -> Voltage Loop/3(Vo 24V)
  Fbk Sel/1 -> Voltage Loop/4(Fbk Sel)
  Current Loop/1(Fixed Pulses) -> Loop Select/1(Fixed Pulses Voltage Loop)
  Current Loop/2(Variable Pulses) -> Loop Select/2(Variable Pulses Volatge Loop)
  Current Loop/3(OverCurrent Status) -> Loop Select/3(OverCurrent Status)
  Voltage Loop/1(Fixed Pulses) -> Loop Select/4(Fixed Pulses Current Loop)
  Voltage Loop/2(Variable Pulses) -> Loop Select/5(Variable Pulses Current Loop)
  Loop Select/1(Fixed Pulses) -> Fixed Pulses/1
  Loop Select/2(Variable Pulses) -> Variable Pulses/1
  Vi/1 -> Voltage Loop/1(Vi)

== system Monorail_Auxiliary_Power_Unit/First Stage/Shared Leg Rectifier 24V ==
  Diode{,1..5} (6 alike) : spsDiodeLib/Diode  Ron=0.001  Lon=0  Vf=0.8  IC=0  UseSnubber=0  Rs=500  Cs=250e-9  Measurements=on
  Scope{1..6} (6 alike) : Scope  Commented=on
  R : PMIOPort  Side=Left
  Y : PMIOPort  Port=2  Side=Left
  B : PMIOPort  Port=3  Side=Left
  +ve : PMIOPort  Port=4  Side=Right
  -ve : PMIOPort  Port=5  Side=Right
  wires:
  Diode5/1 -> Scope6/1
  Diode4/1 -> Scope4/1
  Diode3/1 -> Scope3/1
  Diode/1 -> Scope2/1
  Diode1/1 -> Scope1/1
  Diode2/1 -> Scope5/1
  connections:
  Diode/LConn1 -- R/RConn1 -- Diode5/RConn1
  -ve/RConn1 -- Diode3/LConn1 -- Diode4/LConn1 -- Diode5/LConn1
  B/RConn1 -- Diode2/LConn1 -- Diode3/RConn1
  +ve/RConn1 -- Diode2/RConn1 -- Diode/RConn1 -- Diode1/RConn1
  Y/RConn1 -- Diode1/LConn1 -- Diode4/RConn1

== system Monorail_Auxiliary_Power_Unit/First Stage/Shared Leg Rectifier 750V ==
  Diode{,1..5} (6 alike) : spsDiodeLib/Diode  Ron=0.001  Lon=0  Vf=0.8  IC=0  UseSnubber=0  Rs=500  Cs=250e-9  Measurements=on
  Scope{1..6} (6 alike) : Scope  Commented=on
  R : PMIOPort  Side=Left
  Y : PMIOPort  Port=2  Side=Left
  B : PMIOPort  Port=3  Side=Left
  +ve : PMIOPort  Port=4  Side=Right
  -ve : PMIOPort  Port=5  Side=Right
  wires:
  Diode2/1 -> Scope5/1
  Diode1/1 -> Scope1/1
  Diode/1 -> Scope2/1
  Diode3/1 -> Scope3/1
  Diode4/1 -> Scope4/1
  Diode5/1 -> Scope6/1
  connections:
  Diode4/RConn1 -- Y/RConn1 -- Diode1/LConn1
  Diode2/RConn1 -- Diode1/RConn1 -- Diode/RConn1 -- +ve/RConn1
  Diode3/RConn1 -- B/RConn1 -- Diode2/LConn1
  Diode5/LConn1 -- Diode3/LConn1 -- -ve/RConn1 -- Diode4/LConn1
  Diode5/RConn1 -- R/RConn1 -- Diode/LConn1

== system Monorail_Auxiliary_Power_Unit/First Stage/Variable PSFB ==
  Pulses : Inport
  Demux : Demux  Outputs=2
  IGBT/Diode{,1..3} (4 alike) : spsIGBTDiodeLib/IGBT//Diode  Ron=1e-3  Rs=1e5  Cs=inf  Measurements=on
  Scope{1..3,5} (4 alike) : Scope  Commented=on
  +ve : PMIOPort  Side=Left
  -ve : PMIOPort  Port=2  Side=Left
  Line : PMIOPort  Port=3  Side=Right
  Neutral : PMIOPort  Port=4  Side=Right
  wires:
  IGBT/Diode3/1 -> Scope3/1
  IGBT/Diode2/1 -> Scope2/1
  IGBT/Diode1/1 -> Scope1/1
  IGBT/Diode/1 -> Scope5/1
  Pulses/1 -> Demux/1
  Demux/2 -> [YTop]
  Demux/1 -> [RTop]
  [YTop] -> IGBT/Diode2/1
  [YTop] -> IGBT/Diode1/1
  [RTop] -> IGBT/Diode3/1
  [RTop] -> IGBT/Diode/1
  connections:
  -ve/RConn1 -- IGBT/Diode3/RConn1 -- IGBT/Diode1/RConn1
  IGBT/Diode2/LConn1 -- +ve/RConn1 -- IGBT/Diode/LConn1
  IGBT/Diode1/LConn1 -- Line/RConn1 -- IGBT/Diode/RConn1
  IGBT/Diode3/LConn1 -- Neutral/RConn1 -- IGBT/Diode2/RConn1

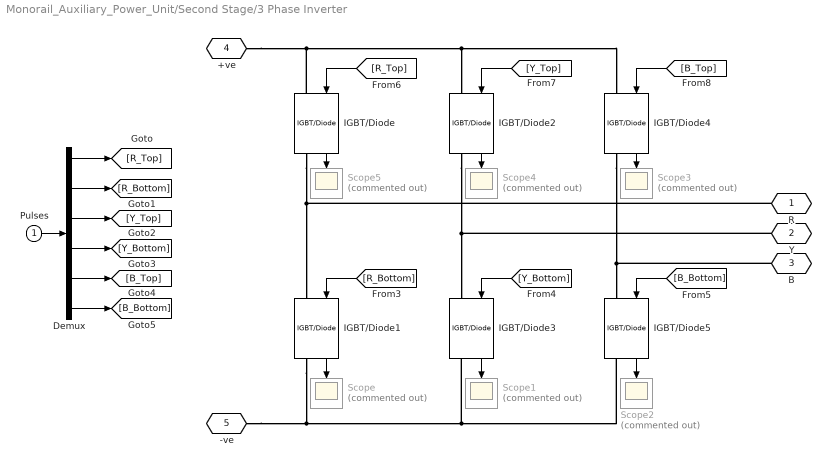
== system Monorail_Auxiliary_Power_Unit/Second Stage/3 Phase Inverter ==
  Pulses : Inport
  Demux : Demux  Outputs=6
  IGBT/Diode{,1..5} (6 alike) : spsIGBTDiodeLib/IGBT//Diode  Ron=1e-3  Rs=1e5  Cs=inf  Measurements=on
  Scope{,1..5} (6 alike) : Scope  Commented=on
  R : PMIOPort  Side=Left
  Y : PMIOPort  Port=2  Side=Left
  B : PMIOPort  Port=3  Side=Left
  +ve : PMIOPort  Port=4  Side=Right
  -ve : PMIOPort  Port=5  Side=Right
  wires:
  [R_Top] -> IGBT/Diode/1
  Pulses/1 -> Demux/1
  Demux/1 -> [R_Top]
  Demux/2 -> [R_Bottom]
  Demux/3 -> [Y_Top]
  Demux/4 -> [Y_Bottom]
  Demux/5 -> [B_Top]
  Demux/6 -> [B_Bottom]
  [R_Bottom] -> IGBT/Diode1/1
  [Y_Top] -> IGBT/Diode2/1
  [Y_Bottom] -> IGBT/Diode3/1
  [B_Top] -> IGBT/Diode4/1
  [B_Bottom] -> IGBT/Diode5/1
  IGBT/Diode/1 -> Scope5/1
  IGBT/Diode1/1 -> Scope/1
  IGBT/Diode3/1 -> Scope1/1
  IGBT/Diode5/1 -> Scope2/1
  IGBT/Diode2/1 -> Scope4/1
  IGBT/Diode4/1 -> Scope3/1
  connections:
  IGBT/Diode4/RConn1 -- IGBT/Diode5/LConn1 -- B/RConn1
  IGBT/Diode2/RConn1 -- IGBT/Diode3/LConn1 -- Y/RConn1
  IGBT/Diode/RConn1 -- R/RConn1 -- IGBT/Diode1/LConn1
  IGBT/Diode/LConn1 -- +ve/RConn1 -- IGBT/Diode2/LConn1 -- IGBT/Diode4/LConn1
  IGBT/Diode1/RConn1 -- IGBT/Diode5/RConn1 -- IGBT/Diode3/RConn1 -- -ve/RConn1

== system Monorail_Auxiliary_Power_Unit/Second Stage/Input Breaker ==
  Enable : Inport
  Breaker : spsBreakerLib/Breaker  InitialState=0  SwitchingTimes="[1/60  5/60]"  External=on  BreakerResistance=0.01  SnubberResistance=1e6  SnubberCapacitance=inf  Measurements=None  MoreParameters=on  NoBreakLoop=off
      settings: SourceProductBaseCode=PS
  Breaker1 : spsBreakerLib/Breaker  InitialState=0  SwitchingTimes="[1/60  5/60]"  External=on  BreakerResistance=0.01  SnubberResistance=1e6  SnubberCapacitance=inf  Measurements=None  MoreParameters=on  NoBreakLoop=off
      settings: SourceProductBaseCode=PS
  +ve In : PMIOPort  Side=Left
  -ve In : PMIOPort  Port=2  Side=Left
  +ve Out : PMIOPort  Port=3  Side=Right
  -ve Out : PMIOPort  Port=4  Side=Right
  wires:
  Enable/1 -> Breaker1/1, Breaker/1
  connections:
  Breaker1/RConn1 -- -ve Out/RConn1
  Breaker1/LConn1 -- -ve In/RConn1
  Breaker/RConn1 -- +ve Out/RConn1
  Breaker/LConn1 -- +ve In/RConn1

== system Monorail_Auxiliary_Power_Unit/Second Stage/Pulse Generator ==
  V feedback : Inport
  I feedback : Inport  Port=2
  Enable : EnablePort
  Current Loop : Subsystem
      settings: PortSchema="{\"entries\":[{\"content\":{\"sides\":[{\"content\":{\"connectorIds\":[\"In1\"]},\"type\":\"ConnectorPlacement.EquallySpacedRectSide\",\"uuid\":\"3301e0b6-592f-4625-8269-e8a7d97e22bd\"},{\"content\":{\"connectorIds\":[\"Out1\",\"Out2\"],\"side\":\"RIGHT\"},\"type\":\"ConnectorPlacement.EquallySpacedRectSide\",\"uuid\":\"054d50bd-24b4-4709-a51e-c662b2406f8c\"},{\"content\":{\"connectorIds\":[],\"side\":\"TOP\"},\"type\":\"ConnectorPlacement.EquallySpacedRectSide\",\"uuid\":\"f115f2c5-740b-4df4-bc67-82446fee67ee\"},{\"content\":{\"connectorIds\":[\"Out3\"],\"side\":\"BOTTOM\"},\"type\":\"ConnectorPlacement.EquallySpacedRectSide\",\"uuid\":\"bf7ffb2f-3623-4d21-9c45-e72b2cab4b93\"}]},\"type\":\"ConnectorPlacement.EquallySpacedConnector\",\"uuid\":\"b1a80dea-a418-49d9-810f-d923c5601f97\"}],\"packageUris\":[\"http://schema.mathworks.com/mf0/Connector/19700101\"],\"version\":\"1.0\"}"
  Deadband : Subsystem
  Loop Select : Subsystem
  Pulse : Subsystem
  Voltage Loop : Subsystem
  Pulses : Outport
  wires:
  Pulse/1(Pulses) -> Deadband/1(Pulses In)
  Deadband/1(Pulses Out) -> Pulses/1
  V feedback/1 -> Voltage Loop/1(V fbk)
  I feedback/1 -> Current Loop/1(I fbk)
  Current Loop/1(I PI Out) -> Loop Select/1(I PI)
  Current Loop/2(I Theta) -> Loop Select/2(I Theta)
  Current Loop/3(Inverter Overcurrent Status) -> Loop Select/3(Inverter Overcurrent Status)
  Voltage Loop/1(V PI Out) -> Loop Select/4(V PI)
  Voltage Loop/2(V Theta) -> Loop Select/5(V Theta)
  Loop Select/1(DQ0) -> Pulse/1(dq0)
  Loop Select/2(Theta) -> Pulse/2(Theta)

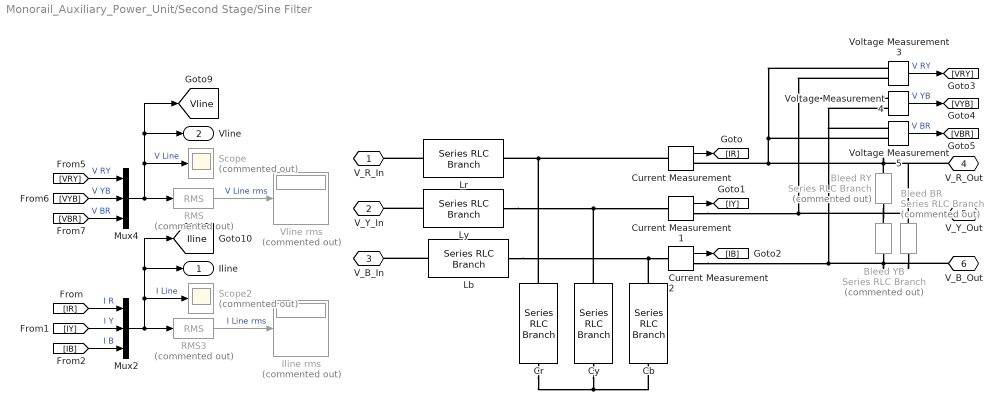
== system Monorail_Auxiliary_Power_Unit/Second Stage/Sine Filter ==
  Bleed BR : spsSeriesRLCBranchLib/Series RLC Branch  Commented=on  LConnTagsString=__new0  RConnTagsString=__new0  BranchType=R  Resistance=1e03  Inductance=1e-3  SetiL0=off  InitialCurrent=0  Capacitance=1e-6  Setx0=off  InitialVoltage=0  Measurements=None
  Bleed RY : spsSeriesRLCBranchLib/Series RLC Branch  Commented=on  LConnTagsString=__new0  RConnTagsString=__new0  BranchType=R  Resistance=1e03  Inductance=1e-3  SetiL0=off  InitialCurrent=0  Capacitance=1e-6  Setx0=off  InitialVoltage=0  Measurements=None
  Bleed YB : spsSeriesRLCBranchLib/Series RLC Branch  Commented=on  LConnTagsString=__new0  RConnTagsString=__new0  BranchType=R  Resistance=1e03  Inductance=1e-3  SetiL0=off  InitialCurrent=0  Capacitance=1e-6  Setx0=off  InitialVoltage=0  Measurements=None
  Cb : spsSeriesRLCBranchLib/Series RLC Branch  LConnTagsString=__new0  RConnTagsString=__new0  BranchType=C  Resistance=1  Inductance=0.85e-3  SetiL0=off  InitialCurrent=0  Capacitance=C_sin_filt  Setx0=off  InitialVoltage=0  Measurements=Branch current
  Cr : spsSeriesRLCBranchLib/Series RLC Branch  LConnTagsString=__new0  RConnTagsString=__new0  BranchType=C  Resistance=1  Inductance=0.85e-3  SetiL0=off  InitialCurrent=0  Capacitance=C_sin_filt  Setx0=off  InitialVoltage=0  Measurements=Branch current
  Current Measurement : spsCurrentMeasurementLib/Current Measurement  PhasorSimulation=off  OutputType=Complex  PSBequivalent=0
  Current Measurement1 : spsCurrentMeasurementLib/Current Measurement  PhasorSimulation=off  OutputType=Complex  PSBequivalent=0
  Current Measurement2 : spsCurrentMeasurementLib/Current Measurement  PhasorSimulation=off  OutputType=Complex  PSBequivalent=0
  Cy : spsSeriesRLCBranchLib/Series RLC Branch  LConnTagsString=__new0  RConnTagsString=__new0  BranchType=C  Resistance=1  Inductance=0.85e-3  SetiL0=off  InitialCurrent=0  Capacitance=C_sin_filt  Setx0=off  InitialVoltage=0  Measurements=Branch current
  Iline rms : Display  Commented=on
  Lb : spsSeriesRLCBranchLib/Series RLC Branch  LConnTagsString=__new0  RConnTagsString=__new0  BranchType=L  Resistance=1  Inductance=L_sin_filt  SetiL0=off  InitialCurrent=0  Capacitance=1e-6  Setx0=off  InitialVoltage=0  Measurements=Branch voltage
  Lr : spsSeriesRLCBranchLib/Series RLC Branch  LConnTagsString=__new0  RConnTagsString=__new0  BranchType=L  Resistance=1  Inductance=L_sin_filt  SetiL0=off  InitialCurrent=0  Capacitance=1e-6  Setx0=off  InitialVoltage=0  Measurements=Branch voltage
  Ly : spsSeriesRLCBranchLib/Series RLC Branch  LConnTagsString=__new0  RConnTagsString=__new0  BranchType=L  Resistance=1  Inductance=L_sin_filt  SetiL0=off  InitialCurrent=0  Capacitance=1e-6  Setx0=off  InitialVoltage=0  Measurements=Branch voltage
  Mux2 : Mux  Inputs=3
  Mux4 : Mux  Inputs=3
  RMS : spsRMSLib/RMS  Commented=on  TrueRMS=on  Freq=50  RMSInit=0  Ts=0
  RMS3 : spsRMSLib/RMS  Commented=on  TrueRMS=on  Freq=50  RMSInit=0  Ts=0
  Scope : Scope  Commented=on
  Scope2 : Scope  Commented=on
  Vline rms : Display  Commented=on
  Voltage Measurement3 : spsVoltageMeasurementLib/Voltage Measurement  PhasorSimulation=off  OutputType=Complex  PSBequivalent=0
  Voltage Measurement4 : spsVoltageMeasurementLib/Voltage Measurement  PhasorSimulation=off  OutputType=Complex  PSBequivalent=0
  Voltage Measurement5 : spsVoltageMeasurementLib/Voltage Measurement  PhasorSimulation=off  OutputType=Complex  PSBequivalent=0
  V_R_In : PMIOPort  Side=Left
  V_Y_In : PMIOPort  Port=2  Side=Left
  V_B_In : PMIOPort  Port=3  Side=Left
  V_R_Out : PMIOPort  Port=4  Side=Right
  V_Y_Out : PMIOPort  Port=5  Side=Right
  V_B_Out : PMIOPort  Port=6  Side=Right
  Iline : Outport
  Vline : Outport  Port=2
  tag scope: Iline=global, Vline=global
  wires:
  Voltage Measurement5/1 -> [VBR]  "V BR"
  Voltage Measurement4/1 -> [VYB]  "V YB"
  RMS/1 -> Vline rms/1  "V Line rms"
  Mux2/1 -> Iline/1, [Iline], Scope2/1, RMS3/1  "I Line"
  RMS3/1 -> Iline rms/1  "I Line rms"
  Voltage Measurement3/1 -> [VRY]  "V RY"
  [IR] -> Mux2/1  "I R"
  [IB] -> Mux2/3  "I B"
  [IY] -> Mux2/2  "I Y"
  Current Measurement/1 -> [IR]
  Current Measurement1/1 -> [IY]
  Current Measurement2/1 -> [IB]
  Mux4/1 -> RMS/1, [Vline], Vline/1, Scope/1  "V Line"
  [VRY] -> Mux4/1  "V RY"
  [VYB] -> Mux4/2  "V YB"
  [VBR] -> Mux4/3  "V BR"
  connections:
  Bleed BR/RConn1 -- V_R_Out/RConn1 -- Bleed RY/LConn1 -- Voltage Measurement3/LConn1 -- Voltage Measurement5/LConn2 -- Current Measurement/RConn1
  Current Measurement2/RConn1 -- Bleed BR/LConn1 -- V_B_Out/RConn1 -- Bleed YB/RConn1 -- Voltage Measurement5/LConn1 -- Voltage Measurement4/LConn2
  Current Measurement1/RConn1 -- Bleed RY/RConn1 -- V_Y_Out/RConn1 -- Bleed YB/LConn1 -- Voltage Measurement4/LConn1 -- Voltage Measurement3/LConn2
  Lr/LConn1 -- V_R_In/RConn1
  Ly/LConn1 -- V_Y_In/RConn1
  Lb/LConn1 -- V_B_In/RConn1
  Ly/RConn1 -- Cy/LConn1 -- Current Measurement1/LConn1
  Lb/RConn1 -- Cb/LConn1 -- Current Measurement2/LConn1
  Current Measurement/LConn1 -- Lr/RConn1 -- Cr/LConn1
  Cr/RConn1 -- Cy/RConn1 -- Cb/RConn1

== system Monorail_Auxiliary_Power_Unit/First Stage/DC Filter 700V/Chopper ==
  Constant : Constant  Value=800
  Constant1 : Constant  Value=10
  Demux : Demux  Outputs=3
  GreaterThan : RelationalOperator  Operator=>  OutDataTypeStr=boolean  RndMeth=Simplest
  GreaterThan1 : RelationalOperator  Operator=<  OutDataTypeStr=boolean  RndMeth=Simplest
  Logical Operator : Logic  IconShape=distinctive  AllPortsSameDT=off  OutDataTypeStr=boolean
  RMS2 : powerlib_meascontrol/Measurements/RMS  TrueRMS=on  Freq=f_fund  RMSInit=0  Ts=0
  Terminator : Terminator
  Terminator1 : Terminator
  Chopper Pulse : Outport
  wires:
  Constant/1 -> GreaterThan/2
  [Vo700] -> GreaterThan/1
  Demux/1 -> RMS2/1
  Constant1/1 -> GreaterThan1/2
  GreaterThan/1 -> Logical Operator/1
  GreaterThan1/1 -> Logical Operator/2
  Demux/3 -> Terminator/1
  Demux/2 -> Terminator1/1
  [Vline] -> Demux/1
  Logical Operator/1 -> Chopper Pulse/1
  RMS2/1 -> GreaterThan1/1

== system Monorail_Auxiliary_Power_Unit/First Stage/PSFB Pulse Generator/Current Loop ==
  Ibat : Inport
  Carrier Wave Generator : Subsystem
  Close Loop : Subsystem
  Comparator : Subsystem
  Modulating Wave Generator : Subsystem
  Pulses for Fixed PSFB : Subsystem
  Pulses for Variable PSFB : Subsystem
  Scope1 : Scope  NumInputPorts=2
  Fixed Pulses : Outport
  Variable Pulses : Outport  Port=2
  OverCurrent Status : Outport  Port=3
  wires:
  Comparator/2(Variable PSFB R Top Pulse) -> Pulses for Variable PSFB/1(Fixed PSFB R Top Pulse)
  Comparator/1(Fixed PSFB R Top Pulse) -> Pulses for Fixed PSFB/1(Fixed PSFB R Top Pulse)
  Pulses for Fixed PSFB/1(Fixed Pulses) -> Fixed Pulses/1, Scope1/1
  Pulses for Variable PSFB/1(Fixed Pulses) -> Variable Pulses/1, Scope1/2
  Carrier Wave Generator/1(Carrier Wave) -> Comparator/1(Carrier Wave)
  Ibat/1 -> Close Loop/1(Ibat)
  Close Loop/2(OverCurrent Status) -> OverCurrent Status/1
  Close Loop/1(Duty) -> Modulating Wave Generator/1(Duty)
  Modulating Wave Generator/1(Fixed Modulating Wave) -> Comparator/2(Fixed Modulating Wave)
  Modulating Wave Generator/2(Variable Modulating Wave) -> Comparator/3(Variable Modulating Wave)
